simulink model "SSSC_PODcontrol"  (R2018a)
settings: Solver=ode23tb  StartTime=0  StopTime=5  MaxStep=1/60  RelTol=1e-4  AbsTol=1e-3
PreLoadFcn:
  | global Kp
  | global Tw
  | global T1
  | global T2
  | global T3
  | global T4
  | %--------------------------------------
  | global Kp1
  | global Tw1
  | global T11
  | global T21
  | global T31
  | global T41
  | %-------------------------------------
  | global Kp2
  | global Tw2
  | global T12
  | global T22
  | global T32
  | global T42
  | %-------------------------------------
InitFcn:
  | global Kp
  | global Tw
  | global T1
  | global T2
  | global T3
  | global T4
  | %--------------------------------------
  | global Kp1
  | global Tw1
  | global T11
  | global T21
  | global T31
  | global T41
  | %-------------------------------------
  | global Kp2
  | global Tw2
  | global T12
  | global T22
  | global T32
  | global T42
  | %-------------------------------------
values from neighbouring files (symbols this model uses):
  Kp = (x(1))    [fitnessfunc.m]
  Kp1 = (x(7))    [fitnessfunc.m]
  Kp2 = (x(13))    [fitnessfunc.m]
  T1 = best_Value(3)    [ACOMain.m]    (also in FPGA_POD_coefficients.mat = 0.46; Main.m; fitnessfunc.m = (x(3)); optimized_POD_parameters.mat = 0.46)
  T11 = (x(9))    [fitnessfunc.m]
  T12 = (x(15))    [fitnessfunc.m]
  T2 = best_Value(4)    [ACOMain.m]    (also in FPGA_POD_coefficients.mat = 0.49; Main.m; fitnessfunc.m = (x(4)); optimized_POD_parameters.mat = 0.49)
  T21 = (x(10))    [fitnessfunc.m]
  T22 = (x(16))    [fitnessfunc.m]
  T3 = best_Value(5)    [ACOMain.m]    (also in FPGA_POD_coefficients.mat = 0.32; Main.m; fitnessfunc.m = (x(5)); optimized_POD_parameters.mat = 0.32)
  T31 = (x(11))    [fitnessfunc.m]
  T32 = (x(17))    [fitnessfunc.m]
  T4 = best_Value(6)    [ACOMain.m]    (also in FPGA_POD_coefficients.mat = 0.1564; Main.m; fitnessfunc.m = (x(6)); optimized_POD_parameters.mat = 0.1564)
  T41 = (x(12))    [fitnessfunc.m]
  T42 = (x(18))    [fitnessfunc.m]
  Tw = best_Value(2)    [ACOMain.m]    (also in FPGA_POD_coefficients.mat = 10.1; Main.m; fitnessfunc.m = (x(2)); optimized_POD_parameters.mat = 10.1)
undefined symbols (not defined in the file or in its folder): D1, Delta
libraries: powerlib x21, powerlib_meascontrol x9, sps_avr x2, factslib x1
Description:
  | Copyright 2008-2018 The MathWorks, Inc.
settings Model: ExtModeAutoUpdateStatusClock=off  Creator=MathWorks  LastModifiedBy=Mehdi
settings SolverCC: AutoScaleAbsTol=off
settings DataIOCC: SaveFinalState=on  SaveFormat=Array  SignalLoggingSaveFormat=ModelDataLogs  SaveOutput=off  SaveTime=off  SignalLoggingName=sigsOut
settings OptimizationCC: BooleanDataType=off  ExpressionDepthLimit=2147483647  InitFltsAndDblsToZero=on  LifeSpan=inf
settings DebuggingCC: UnderspecifiedInitializationDetection=Classic  MergeDetectMultiDrivingBlocksExec=none  CheckExecutionContextPreStartOutputMsg=on  CheckExecutionContextRuntimeOutputMsg=on  SignalResolutionControl=TryResolveAllWithWarning  MultiTaskDSMMsg=warning  MultiTaskCondExecSysMsg=none  SigSpecEnsureSampleTimeMsg=none  FcnCallInpInsideContextMsg=warning  UnconnectedLineMsg=none  StateNameClashWarn=warning  SFUnexpectedBacktrackingDiag=warning  SFNoUnconditionalDefaultTransitionDiag=warning  SFExecutionAtInitializationDiag=none
settings HardwareCC: ProdBitPerPointer=32  ProdBitPerSizeT=32  ProdBitPerPtrDiffT=32  ProdLargestAtomicFloat=None  ProdIntDivRoundTo=Undefined  ProdEndianess=Unspecified  ProdWordSize=32  ProdHWDeviceType=32-bit Generic  TargetUnknown=on
settings ModelReferenceCC: PropagateSignalLabelsOutOfModel=off
settings CodeAppCC: StateflowObjectComments=on
settings GRTTargetCC: TargetLangStandard=C89/C90 (ANSI)  GeneratePreprocessorConditionals=Disable all  CombineOutputUpdateFcns=off  GRTInterface=on
settings ConfigComp: CovMetricSettings=dw  CovHtmlReporting=on  CovSaveCumulativeToWorkspaceVar=on  CovSaveSingleToWorkspaceVar=on  CovExternalEMLEnable=off  CovSFcnEnable=off
settings SimscapeCC: SimscapeNormalizeSystem=off

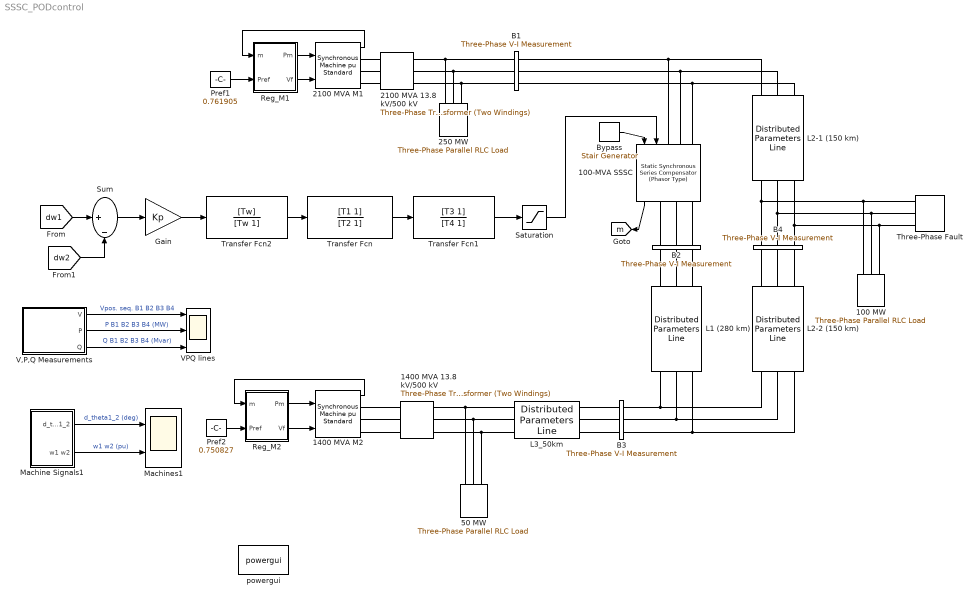
== system SSSC_PODcontrol ==
  100 MW : powerlib/Elements/Three-Phase Parallel RLC Load  LConnTagsString=A|B|C  Configuration=Y (grounded)  NominalVoltage=500e3  Vabc=[1e3 1e3 1e3]  Vabcp=[1e3 1e3 1e3]  NominalFrequency=60  UnbalancedPower=off  ActivePower=100e6  InductivePower=0  CapacitivePower=0  Pabc=[10e3 9e3 11e3]  QLabc=[100 90 110]  QCabc=[100 90 110]  Pabcp=[10e3 9e3 11e3]  QLabcp=[100 90 110]  QCabcp=[100 90 110]  Measurements=None  LoadType=constant Z
  100-MVA SSSC : factslib/Power-Electronics Based FACTS/Static Synchronous Series Compensator (Phasor Type)  SystemNominal=[ 500e3, 60 ]  SeriesNominal=[ 100e6, 0.1]  RL=[ 0.16/30, 0.16 ]  Iinit=[ 0 0]  VnomDC=40000  C_DC=375e-6  ExternalByPass=External control  Vqref=0.05  ExternalVqref=on  MaxRateVqRef=3  Par_VacReg=[0.03 1.5]/8  Par_VdcReg=[0.1e-3 20e-3]
      settings: SourceProductName=Simscape Power Systems  SourceProductBaseCode=PS
  1400 MVA M2 : powerlib/Machines/Synchronous Machine pu Standard  PresetModel=No  MechanicalLoad=Mechanical power Pm  ShowDetailedParameters=on  RotorType=Salient-pole  Units=per unit standard parameters  MeasurementBus=off  NominalParameters="[1400E6  13800   60 ]"  Reactances1=[ 31 32 33 34 35 36 37 ]  Reactances2=[ 1.305, 0.296, 0.252, 0.474, 0.243, 0.18 ]  dAxisTimeConstants=Short-circuit  qAxisTimeConstants=Open-circuit  TimeConstants1=[]  TimeConstants2=[]  TimeConstants3=[]  TimeConstants4=[]  TimeConstants5=[ 1.01, 0.053, 0.1 ]  TimeConstants6=[]  TimeConstants7=[]  TimeConstants8=[]  StatorResistance=2.8544e-3  Mechanical="[ 3.7 0  32]"  PolePairs=32  InitialConditions=[0 -71.2244 0.745111 0.745111 0.745111 -3.89206 -123.892 116.108 1.33295]  SetSaturation=off  Saturation=[0.6404,0.7127,0.8441,0.9214,0.9956,1.082,1.19,1.316,1.457;0.7,0.7698,0.8872,0.9466,0.9969,1.046,1.1,1.151,1.201]  LoadFlowParameters=[2 1000000000 13938 0 0]  TsPowergui=0  TsBlock=-1  IterativeModel=Forward Euler  IterativeDiscreteModel=Trapezoidal non iterative  BusType=PV  Pref=0  Qref=0  Qmin=-inf  Qmax=inf  PLF=0  QLF=0
      settings: AttributesFormatString=\n\n  SourceProductName=Simscape Power Systems
  1400 MVA 13.8 kV/500 kV : powerlib/Elements/Three-Phase Transformer (Two Windings)  Winding1Connection=Delta (D1)  Winding2Connection=Yg  CoreType=Three single-phase transformers  SetSaturation=off  Hysteresis=off  DataFile='basic_model'  SetInitialFlux=off  Measurements=None  UNITS=pu  NominalPower=[ 1400e6 60 ]  Winding1="[ 13.8e3 0.002  0.0]"  Winding2=[ 500e3 0.002 0.12]  Rm=500  Lm=500  L0=0.5  Saturation="[ 0,0  ;  0.005,1.2  ;  1.0,1.4 ]"  InitialFluxes=[ 0.8 , -0.8 , 0.7 ]  MoreParameters=off  BreakLoop=off  DataType=off  TransfoNumber=0
  2100 MVA M1 : powerlib/Machines/Synchronous Machine pu Standard  PresetModel=No  MechanicalLoad=Mechanical power Pm  ShowDetailedParameters=on  RotorType=Salient-pole  Units=per unit standard parameters  MeasurementBus=off  NominalParameters="[2100E6  13800   60 ]"  Reactances1=[ 31 32 33 34 35 36 37 ]  Reactances2=[ 1.305, 0.296, 0.252, 0.474, 0.243, 0.18 ]  dAxisTimeConstants=Short-circuit  qAxisTimeConstants=Open-circuit  TimeConstants1=[]  TimeConstants2=[]  TimeConstants3=[]  TimeConstants4=[]  TimeConstants5=[ 1.01, 0.053, 0.1 ]  TimeConstants6=[]  TimeConstants7=[]  TimeConstants8=[]  StatorResistance=2.8544e-3  Mechanical="[ 3.7 0  32]"  PolePairs=32  InitialConditions=[0 -58.9841 0.763417 0.763417 0.763417 14.3746 -105.625 134.375 1.2256]  SetSaturation=off  Saturation=[0.6404,0.7127,0.8441,0.9214,0.9956,1.082,1.19,1.316,1.457;0.7,0.7698,0.8872,0.9466,0.9969,1.046,1.1,1.151,1.201]  LoadFlowParameters=[1 1600000000 0 0 0]  TsPowergui=0  TsBlock=-1  IterativeModel=Forward Euler  IterativeDiscreteModel=Trapezoidal non iterative  BusType=PV  Pref=0  Qref=0  Qmin=-inf  Qmax=inf  PLF=0  QLF=0
      settings: AttributesFormatString=\n\n  SourceProductName=Simscape Power Systems
  2100 MVA 13.8 kV/500 kV : powerlib/Elements/Three-Phase Transformer (Two Windings)  Winding1Connection=Delta (D1)  Winding2Connection=Yg  CoreType=Three single-phase transformers  SetSaturation=off  Hysteresis=off  DataFile='basic_model'  SetInitialFlux=off  Measurements=None  UNITS=pu  NominalPower=[ 2100e6 60 ]  Winding1="[ 13.8e3 0.002  0.0]"  Winding2=[ 500e3 0.002 0.12]  Rm=500  Lm=500  L0=0.5  Saturation="[ 0,0  ;  0.005,1.2  ;  1.0,1.4 ]"  InitialFluxes=[ 0.8 , -0.8 , 0.7 ]  MoreParameters=off  BreakLoop=off  DataType=off  TransfoNumber=0
  250 MW : powerlib/Elements/Three-Phase Parallel RLC Load  LConnTagsString=A|B|C  Configuration=Y (grounded)  NominalVoltage=500e3  Vabc=[1e3 1e3 1e3]  Vabcp=[1e3 1e3 1e3]  NominalFrequency=60  UnbalancedPower=off  ActivePower=250e6  InductivePower=0  CapacitivePower=0  Pabc=[10e3 9e3 11e3]  QLabc=[100 90 110]  QCabc=[100 90 110]  Pabcp=[10e3 9e3 11e3]  QLabcp=[100 90 110]  QCabcp=[100 90 110]  Measurements=None  LoadType=constant Z
  50 MW : powerlib/Elements/Three-Phase Parallel RLC Load  LConnTagsString=A|B|C  Configuration=Y (grounded)  NominalVoltage=500e3  Vabc=[1e3 1e3 1e3]  Vabcp=[1e3 1e3 1e3]  NominalFrequency=60  UnbalancedPower=off  ActivePower=50e6  InductivePower=0  CapacitivePower=0  Pabc=[10e3 9e3 11e3]  QLabc=[100 90 110]  QCabc=[100 90 110]  Pabcp=[10e3 9e3 11e3]  QLabcp=[100 90 110]  QCabcp=[100 90 110]  Measurements=None  LoadType=constant Z
  B1 : powerlib/Measurements/Three-Phase V-I Measurement  VoltageMeasurement=phase-to-ground  SetLabelV=on  LabelV=Vabc_B1  Vpu=on  VpuLL=off  CurrentMeasurement=yes  SetLabelI=on  LabelI=Iabc_B1  Ipu=on  Pbase=100e6  Vbase=500e3  OutputType=Complex  PhasorSimulation=on  PSBequivalent=0
  B2 : powerlib/Measurements/Three-Phase V-I Measurement  VoltageMeasurement=phase-to-ground  SetLabelV=on  LabelV=Vabc_B2  Vpu=on  VpuLL=off  CurrentMeasurement=yes  SetLabelI=on  LabelI=Iabc_B2  Ipu=on  Pbase=100e6  Vbase=500e3  OutputType=Complex  PhasorSimulation=on  PSBequivalent=0
  B3 : powerlib/Measurements/Three-Phase V-I Measurement  VoltageMeasurement=phase-to-ground  SetLabelV=on  LabelV=Vabc_B3  Vpu=on  VpuLL=off  CurrentMeasurement=yes  SetLabelI=on  LabelI=Iabc_B3  Ipu=on  Pbase=100e6  Vbase=500e3  OutputType=Complex  PhasorSimulation=on  PSBequivalent=0
  B4 : powerlib/Measurements/Three-Phase V-I Measurement  VoltageMeasurement=phase-to-ground  SetLabelV=on  LabelV=Vabc_B4  Vpu=on  VpuLL=off  CurrentMeasurement=yes  SetLabelI=on  LabelI=Iabc_B4  Ipu=on  Pbase=100e6  Vbase=500e3  OutputType=Complex  PhasorSimulation=on  PSBequivalent=0
  Bypass : powerlib_meascontrol/Pulse & Signal Generators/Stair Generator  t=[0, 0.1]  e=[1, 0 ]  Ts=0
      settings: SourceProductName=Simscape Power Systems
  Gain : Gain  Gain=Kp
  L1 (280 km) : powerlib/Elements/Distributed Parameters Line  Phases=3  Frequency=60  Resistance=[0.01273*2 0.3864]  Inductance="[0.9337e-3  4.1264e-3]"  Capacitance=[12.74e-9 7.751e-9]  Length=280  x1=[8.57453623118534e-09 1498726.92101237 1498731.61187745;376.991118430775 376.991118430775 376.991118430775;-0.207010743951092 -0.27921503857041 -1.85001560704433]  x2=[3.70968821408053e-08 1547199.03240546 1547203.81684282;376.991118430775 376.991118430775 376.991118430775;-1.73289441680718 -0.258096765893564 -1.8288976303327]  x3=[7.34085838580846e-11 5978.20234022193 5978.21644518815;376.991118430775 376.991118430775 376.991118430775;3.00344553485436 -0.528094897252935 -2.09889563309672]  x4=[8.19150865277484e-11 5275.11122531886 5275.13210158224;376.991118430775 376.991118430775 376.991118430775;-0.77313679488924 -0.365166148081062 -1.93596698668438]  x5=0.00158351638758808  V1=ones(3,3)  V2=ones(3,3)  I1=ones(3,3)  I2=ones(3,3)  nHarmo=1  Measurements=None
      settings: AttributesFormatString=\n  SourceProductName=Simscape Power Systems
  L2-1 (150 km) : powerlib/Elements/Distributed Parameters Line  Phases=3  Frequency=60  Resistance=[0.01273*2 0.3864]  Inductance="[0.9337e-3  4.1264e-3]"  Capacitance=[12.74e-9 7.751e-9]  Length=150  x1=[8.14603489907096e-09 1498726.88392124 1498731.57478671;376.991118430775 376.991118430775 376.991118430775;-1.17916675081451 -0.110185299814799 -1.68098586828873]  x2=[1.43076082998811e-07 1551001.48715857 1551006.3144557;376.991118430775 376.991118430775 376.991118430775;-1.56135800434571 -0.111564642343529 -1.68236536135358]  x3=[5.49715704458232e-10 5715.20612101038 5715.21968310763;376.991118430775 376.991118430775 376.991118430775;-2.89588916944808 -0.380270362847911 -1.95107110411091]  x4=[5.12825351090249e-10 5653.45328530216 5653.47513824224;376.991118430775 376.991118430775 376.991118430775;-0.12404020965703 -0.0353350035895054 -1.60613581272854]  x5=0.000848312350493614  V1=ones(3,3)  V2=ones(3,3)  I1=ones(3,3)  I2=ones(3,3)  nHarmo=1  Measurements=None
      settings: AttributesFormatString=\n  SourceProductName=Simscape Power Systems
  L2-2 (150 km) : powerlib/Elements/Distributed Parameters Line  Phases=3  Frequency=60  Resistance=[0.01273*2 0.3864]  Inductance="[0.9337e-3  4.1264e-3]"  Capacitance=[12.74e-9 7.751e-9]  Length=150  x1=[1.43076082998811e-07 1551001.48715857 1551006.3144557;376.991118430775 376.991118430775 376.991118430775;-1.56135800434571 -0.111564642343529 -1.68236536135358]  x2=[3.70968821408053e-08 1547199.03240546 1547203.81684282;376.991118430775 376.991118430775 376.991118430775;-1.45572902458812 -0.0890671266930067 -1.65986799113215]  x3=[4.05230677949172e-10 6333.0550295995 6333.07045412649;376.991118430775 376.991118430775 376.991118430775;-0.243158405131011 -0.179600649437888 -1.75040138546907]  x4=[4.4859545811629e-10 5046.70981789123 5046.72971787752;376.991118430775 376.991118430775 376.991118430775;-2.82744541099243 -0.221522382170995 -1.79232320866502]  x5=0.000848312350493614  V1=ones(3,3)  V2=ones(3,3)  I1=ones(3,3)  I2=ones(3,3)  nHarmo=1  Measurements=None
      settings: AttributesFormatString=\n  SourceProductName=Simscape Power Systems
  L3_50km : powerlib/Elements/Distributed Parameters Line  Phases=3  Frequency=60  Resistance=[0.01273*2 0.3864]  Inductance="[0.9337e-3  4.1264e-3]"  Capacitance=[12.74e-9 7.751e-9]  Length=50  x1=[3.70968821408053e-08 1547199.03240546 1547203.81684282;376.991118430775 376.991118430775 376.991118430775;-1.2425248767273 0.0409556726920371 -1.5298451917471]  x2=[1.70902936205603e-09 1523504.65927186 1523509.34411468;376.991118430775 376.991118430775 376.991118430775;-0.382562555915443 0.0539283570396382 -1.51687260959561]  x3=[4.3479436689631e-10 6826.59857622228 6826.61106408169;376.991118430775 376.991118430775 376.991118430775;0.404606683004551 0.223538538849403 -1.34726198288477]  x4=[4.43312318202334e-10 4841.29117916682 4841.31490602355;376.991118430775 376.991118430775 376.991118430775;-2.61441187928109 -0.281614140729434 -1.85241468519146]  x5=0.000282770783497871  V1=ones(3,3)  V2=ones(3,3)  I1=ones(3,3)  I2=ones(3,3)  nHarmo=1  Measurements=None
      settings: AttributesFormatString=\n  SourceProductName=Simscape Power Systems
  Machine Signals1 : Subsystem
  Machines1 : Scope  NumInputPorts=2
  Pref1 : Constant  Value=0.761905
  Pref2 : Constant  Value=0.750827
  Reg_M1 : Subsystem
  Reg_M2 : Subsystem
  Saturation : Saturate  UpperLimit=0.15  LowerLimit=-0.15
  Sum : Sum  Inputs=|+-
  Three-Phase Fault : powerlib/Elements/Three-Phase Fault  InitialStates=0  FaultA=off  FaultB=off  FaultC=off  GroundFault=on  SwitchTimes=[ 20/60 30/60]+1  External=off  SwitchStatus=NaN  FaultResistance=0.001  GroundResistance=0.001  SnubberResistance=1e6  SnubberCapacitance=inf  Measurements=None
  Transfer Fcn : TransferFcn  Numerator=[T1 1]  Denominator=[T2 1]
  Transfer Fcn1 : TransferFcn  Numerator=[T3 1]  Denominator=[T4 1]
  Transfer Fcn2 : TransferFcn  Numerator=[Tw]  Denominator=[Tw 1]
  V,P,Q Measurements : Subsystem
      mask Display: disp('V P Q\nMeasurements')
  VPQ lines : Scope  NumInputPorts=3
  powergui : powerlib/powergui  Priority=2  SimulationMode=Phasor  SampleTime=0  frequency=60  Iterations=50  frequencyindice=60  Pbase=100e6  ErrMax=1e-4  UnitsV=kV  UnitsW=MW  buscounter=0  FunctionMessages=off  echomessages=off  EnableUseOfTLC=off  CurrentSourceSwitches=off  DisableSnubberDevices=off  DisableRonSwitches=off  DisableVfSwitches=off  DisplayEquations=off  SolverType=Tustin  Interpol=off  ExternalGateDelay=off  methode=off  Ts=0  x0status=blocks  SPID=off  SwTol=0  HookPort=off  RestoreLinks=warning  ResistiveCurrentMeasurement=off  Frange=[0:2:500]  Ylog=off  Xlog=on  ShowGrid=off  save=off  variable=ZData  structure=0  ZoomFFT=on  StartTime=0.0  cycles=1  DisplayStyle=1  fundamental=60  FreqAxis=off  MaxFrequency=1000  frequencyindicesteady=1  RmsSteady=1  display=off
  tag scope: m=global
  wires:
  Reg_M1/1(Pm) -> 2100 MVA M1/1
  Reg_M1/2(Vf) -> 2100 MVA M1/2
  Pref1/1 -> Reg_M1/2(Pref)
  2100 MVA M1/1 -> Reg_M1/1(m)
  Reg_M2/1(Pm) -> 1400 MVA M2/1
  Reg_M2/2(Vf) -> 1400 MVA M2/2
  Pref2/1 -> Reg_M2/2(Pref)
  1400 MVA M2/1 -> Reg_M2/1(m)
  100-MVA SSSC/1 -> [m]
  Bypass/1 -> 100-MVA SSSC/1
  Transfer Fcn/1 -> Transfer Fcn1/1
  Gain/1 -> Transfer Fcn2/1
  Transfer Fcn2/1 -> Transfer Fcn/1
  Sum/1 -> Gain/1
  [dw2] -> Sum/2
  [dw1] -> Sum/1
  Transfer Fcn1/1 -> Saturation/1
  Saturation/1 -> 100-MVA SSSC/2
  V,P,Q Measurements/3(Q) -> VPQ lines/3  "Q B1 B2 B3 B4 (Mvar)"
  V,P,Q Measurements/2(P) -> VPQ lines/2  "P B1 B2 B3 B4 (MW)"
  Machine Signals1/2(w1 w2) -> Machines1/2  "w1 w2 (pu)"
  V,P,Q Measurements/1(V) -> VPQ lines/1  "Vpos. seq. B1 B2 B3 B4"
  Machine Signals1/1(d_theta1_2) -> Machines1/1  "d_theta1_2 (deg)"
  connections:
  2100 MVA M1/RConn1 -- 2100 MVA 13.8 kV/500 kV/LConn1
  2100 MVA M1/RConn2 -- 2100 MVA 13.8 kV/500 kV/LConn2
  2100 MVA M1/RConn3 -- 2100 MVA 13.8 kV/500 kV/LConn3
  250 MW/LConn1 -- 2100 MVA 13.8 kV/500 kV/RConn1 -- B1/LConn1
  250 MW/LConn2 -- 2100 MVA 13.8 kV/500 kV/RConn2 -- B1/LConn2
  250 MW/LConn3 -- 2100 MVA 13.8 kV/500 kV/RConn3 -- B1/LConn3
  100-MVA SSSC/LConn1 -- B1/RConn1 -- L2-1 (150 km)/LConn1
  100-MVA SSSC/LConn2 -- B1/RConn2 -- L2-1 (150 km)/LConn2
  100-MVA SSSC/LConn3 -- B1/RConn3 -- L2-1 (150 km)/LConn3
  1400 MVA M2/RConn1 -- 1400 MVA 13.8 kV/500 kV/LConn1
  1400 MVA M2/RConn2 -- 1400 MVA 13.8 kV/500 kV/LConn2
  1400 MVA M2/RConn3 -- 1400 MVA 13.8 kV/500 kV/LConn3
  B3/RConn1 -- L2-2 (150 km)/RConn1 -- L1 (280 km)/RConn1
  B3/RConn2 -- L2-2 (150 km)/RConn2 -- L1 (280 km)/RConn2
  B3/RConn3 -- L1 (280 km)/RConn3 -- L2-2 (150 km)/RConn3
  B4/RConn1 -- L2-2 (150 km)/LConn1
  B4/RConn2 -- L2-2 (150 km)/LConn2
  B4/RConn3 -- L2-2 (150 km)/LConn3
  Three-Phase Fault/LConn1 -- B4/LConn1 -- L2-1 (150 km)/RConn1 -- 100 MW/LConn1
  Three-Phase Fault/LConn2 -- B4/LConn2 -- L2-1 (150 km)/RConn2 -- 100 MW/LConn2
  Three-Phase Fault/LConn3 -- B4/LConn3 -- L2-1 (150 km)/RConn3 -- 100 MW/LConn3
  1400 MVA 13.8 kV/500 kV/RConn1 -- L3_50km/RConn1 -- 50 MW/LConn1
  1400 MVA 13.8 kV/500 kV/RConn2 -- L3_50km/RConn2 -- 50 MW/LConn2
  1400 MVA 13.8 kV/500 kV/RConn3 -- L3_50km/RConn3 -- 50 MW/LConn3
  100-MVA SSSC/RConn1 -- B2/LConn1
  100-MVA SSSC/RConn2 -- B2/LConn2
  100-MVA SSSC/RConn3 -- B2/LConn3
  B2/RConn1 -- L1 (280 km)/LConn1
  B2/RConn2 -- L1 (280 km)/LConn2
  B2/RConn3 -- L1 (280 km)/LConn3
  L3_50km/LConn1 -- B3/LConn1
  L3_50km/LConn2 -- B3/LConn2
  L3_50km/LConn3 -- B3/LConn3

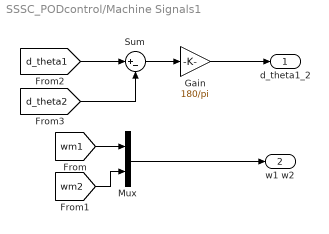
== system SSSC_PODcontrol/Machine Signals1 ==
  Gain : Gain  Gain=180/pi  SaturateOnIntegerOverflow=on  OutDataTypeStr=Inherit: Same as input  ParamDataTypeStr=Inherit: Same as input
  Mux : Mux  Inputs=2
  Sum : Sum  Inputs=|+-  SaturateOnIntegerOverflow=on  InputSameDT=on  OutDataTypeStr=Inherit: Same as first input
  d_theta1_2 : Outport
  w1 w2 : Outport  Port=2
  wires:
  Sum/1 -> Gain/1
  [d_theta1] -> Sum/1
  [wm1] -> Mux/1
  Mux/1 -> w1 w2/1
  Gain/1 -> d_theta1_2/1
  [wm2] -> Mux/2
  [d_theta2] -> Sum/2

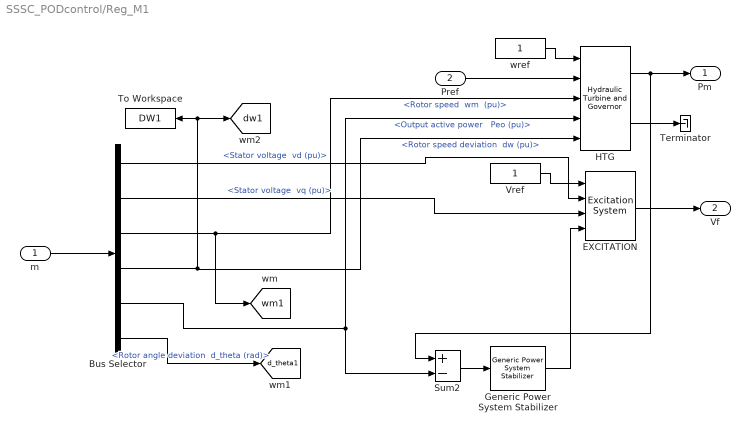
== system SSSC_PODcontrol/Reg_M1 ==
  m : Inport
  Pref : Inport  Port=2
  Bus Selector : BusSelector  OutputSignals="dq0 components.Stator voltage  vd (pu),dq0 components.Stator voltage  vq (pu),Mechanical.Rotor speed  wm  (pu),Mechanical.Rotor speed deviation  dw (pu),Output active power   Peo (pu),Mechanical.Rotor angle deviation  d_theta (rad)"
  EXCITATION : sps_avr/Excitation System  tr=20e-3  reg=[ 200, 0.001 ]  exc=[ 1, 0 ]  tgr=[ 0, 0 ]  damp=[ 0.001, 0.1 ]  sat=[ 0, 0 ]  lim="[ 0,  7, 0 ]"  v0=[1,1.2256]
      settings: SourceProductName=Simscape Power Systems  SourceProductBaseCode=PS
  Generic Power System Stabilizer : powerlib/Machines/Generic Power System Stabilizer  Tsensor=15e-3  K=Kp1  Twashout=Tw1  Tleadlag1=[T11 T21]  Tleadlag2="[T31  T41]"  VSlimits=[-0.15 0.15]  Vinit=0  Plot_On=off  MagdB_On=on  FreqRange=logspace(-2,2,500)
      settings: SourceProductName=Simscape Power Systems  SourceProductBaseCode=PS
  HTG : powerlib/Machines/Hydraulic Turbine and Governor  sm="[ 10/3  0.07 ]"  gate="[  0.01  0.97518  -0.1  0.1 ]"  reg="[  0.05  1.163  0.105  0  0.01  ]"  hyd="[  0  2.67  ]"  dref=0  po=0.763568
      settings: SourceProductName=Simscape Power Systems  SourceProductBaseCode=PS
  Sum2 : Sum  Inputs=+-  SaturateOnIntegerOverflow=on  InputSameDT=on  OutDataTypeStr=Inherit: Same as first input
  Terminator : Terminator
  To Workspace : ToWorkspace  VariableName=DW1  SampleTime=-1
  Vref : Constant
  wref : Constant
  Pm : Outport  InitialOutput=0
  Vf : Outport  Port=2  InitialOutput=0
  tag scope: d_theta1=global, dw1=global, wm1=global
  wires:
  Sum2/1 -> Generic Power System Stabilizer/1
  Bus Selector/1 -> EXCITATION/2  "<Stator voltage  vd (pu)>"
  EXCITATION/1 -> Vf/1
  Bus Selector/2 -> EXCITATION/3  "<Stator voltage  vq (pu)>"
  HTG/1 -> Sum2/1, Pm/1
  wref/1 -> HTG/1
  Pref/1 -> HTG/2
  Bus Selector/3 -> [wm1], HTG/3  "<Rotor speed  wm  (pu)>"
  Bus Selector/5 -> HTG/4, Sum2/2  "<Output active power   Peo (pu)>"
  Bus Selector/4 -> HTG/5, To Workspace/1, [dw1]  "<Rotor speed deviation  dw (pu)>"
  m/1 -> Bus Selector/1
  Vref/1 -> EXCITATION/1
  HTG/2 -> Terminator/1
  Generic Power System Stabilizer/1 -> EXCITATION/4
  Bus Selector/6 -> [d_theta1]  "<Rotor angle deviation  d_theta (rad)>"

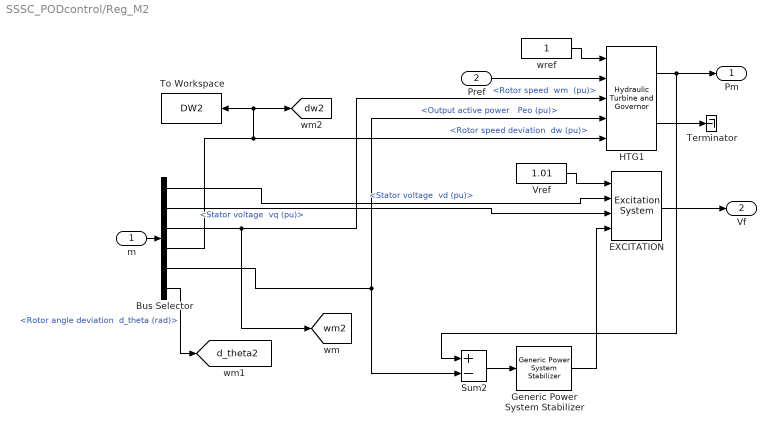
== system SSSC_PODcontrol/Reg_M2 ==
  m : Inport
  Pref : Inport  Port=2
  Bus Selector : BusSelector  OutputSignals="dq0 components.Stator voltage  vd (pu),dq0 components.Stator voltage  vq (pu),Mechanical.Rotor speed  wm  (pu),Mechanical.Rotor speed deviation  dw (pu),Output active power   Peo (pu),Mechanical.Rotor angle deviation  d_theta (rad)"
  EXCITATION : sps_avr/Excitation System  tr=20e-3  reg=[ 200, 0.001 ]  exc=[ 1, 0 ]  tgr=[ 0, 0 ]  damp=[ 0.001, 0.1 ]  sat=[ 0, 0 ]  lim="[ 0,  7, 0 ]"  v0=[1.01,1.33295]
      settings: SourceProductName=Simscape Power Systems  SourceProductBaseCode=PS
  Generic Power System Stabilizer : powerlib/Machines/Generic Power System Stabilizer  Tsensor=15e-3  K=Kp2  Twashout=Tw2  Tleadlag1="[T12  T22]"  Tleadlag2="[T32  T42]"  VSlimits=[-0.15 0.15]  Vinit=0  Plot_On=off  MagdB_On=on  FreqRange=logspace(-2,2,500)
      settings: SourceProductName=Simscape Power Systems  SourceProductBaseCode=PS
  HTG1 : powerlib/Machines/Hydraulic Turbine and Governor  sm="[ 10/3  0.07 ]"  gate="[  0.01  0.97518  -0.1  0.1 ]"  reg="[  0.05  1.163  0.105  0  0.01  ]"  hyd="[  0  2.67  ]"  dref=0  po=0.752412
      settings: SourceProductName=Simscape Power Systems  SourceProductBaseCode=PS
  Sum2 : Sum  Inputs=+-  SaturateOnIntegerOverflow=on  InputSameDT=on  OutDataTypeStr=Inherit: Same as first input
  Terminator : Terminator
  To Workspace : ToWorkspace  VariableName=DW2  SampleTime=-1
  Vref : Constant  Value=1.01
  wref : Constant
  Pm : Outport  InitialOutput=0
  Vf : Outport  Port=2  InitialOutput=0
  tag scope: d_theta2=global, dw2=global, wm2=global
  wires:
  HTG1/2 -> Terminator/1
  Vref/1 -> EXCITATION/1
  m/1 -> Bus Selector/1
  Bus Selector/4 -> HTG1/5, [dw2], To Workspace/1  "<Rotor speed deviation  dw (pu)>"
  Bus Selector/5 -> Sum2/2, HTG1/4  "<Output active power   Peo (pu)>"
  Bus Selector/3 -> [wm2], HTG1/3  "<Rotor speed  wm  (pu)>"
  Pref/1 -> HTG1/2
  wref/1 -> HTG1/1
  HTG1/1 -> Pm/1, Sum2/1
  Bus Selector/2 -> EXCITATION/3  "<Stator voltage  vq (pu)>"
  EXCITATION/1 -> Vf/1
  Bus Selector/1 -> EXCITATION/2  "<Stator voltage  vd (pu)>"
  Sum2/1 -> Generic Power System Stabilizer/1
  Generic Power System Stabilizer/1 -> EXCITATION/4
  Bus Selector/6 -> [d_theta2]  "<Rotor angle deviation  d_theta (rad)>"

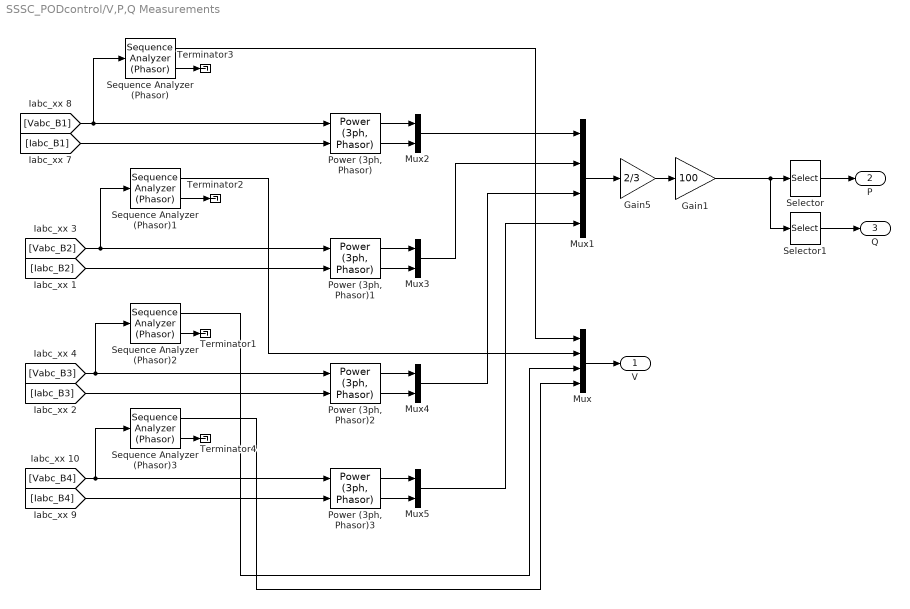
== system SSSC_PODcontrol/V,P,Q Measurements ==
  Gain1 : Gain  Gain=100  SaturateOnIntegerOverflow=on  OutDataTypeStr=Inherit: Same as input  ParamDataTypeStr=Inherit: Same as input
  Gain5 : Gain  Gain=2/3  SaturateOnIntegerOverflow=on  OutDataTypeStr=Inherit: Same as input  ParamDataTypeStr=Inherit: Same as input
  Mux : Mux
  Mux1 : Mux
  Mux{2..5} (4 alike) : Mux  Inputs=2
  Power (3ph, Phasor){,1..3} (4 alike) : powerlib_meascontrol/Measurements/Power (3ph, Phasor)
      settings: SourceProductName=Simscape Power Systems  SourceProductBaseCode=PS
  Selector : Selector  InputPortWidth=8  IndexOptions=Index vector (dialog)  Indices=[1 3 5 7 ]  OutputSizes=1
  Selector1 : Selector  InputPortWidth=8  IndexOptions=Index vector (dialog)  Indices=[1 3 5 7 ]+1  OutputSizes=1
  Sequence Analyzer (Phasor){,1..3} (4 alike) : powerlib_meascontrol/Measurements/Sequence Analyzer (Phasor)  seq=Positive
      settings: SourceProductName=Simscape Power Systems  SourceProductBaseCode=PS
  Terminator{1..4} (4 alike) : Terminator
  V : Outport
  P : Outport  Port=2
  Q : Outport  Port=3
  wires:
  Gain1/1 -> Selector/1, Selector1/1
  Gain5/1 -> Gain1/1
  Sequence Analyzer (Phasor)1/2 -> Terminator2/1
  [Vabc_B2] -> "Power (3ph, Phasor)1"/1, Sequence Analyzer (Phasor)1/1
  [Iabc_B2] -> "Power (3ph, Phasor)1"/2
  [Vabc_B3] -> "Power (3ph, Phasor)2"/1, Sequence Analyzer (Phasor)2/1
  [Iabc_B3] -> "Power (3ph, Phasor)2"/2
  Sequence Analyzer (Phasor)2/2 -> Terminator1/1
  Sequence Analyzer (Phasor)1/1 -> Mux/2
  Sequence Analyzer (Phasor)2/1 -> Mux/3
  Mux/1 -> V/1
  Mux1/1 -> Gain5/1
  Selector/1 -> P/1
  Selector1/1 -> Q/1
  Sequence Analyzer (Phasor)3/2 -> Terminator4/1
  Sequence Analyzer (Phasor)3/1 -> Mux/4
  Sequence Analyzer (Phasor)/1 -> Mux/1
  [Vabc_B1] -> "Power (3ph, Phasor)"/1, Sequence Analyzer (Phasor)/1
  [Iabc_B1] -> "Power (3ph, Phasor)"/2
  "Power (3ph, Phasor)"/2 -> Mux2/2
  "Power (3ph, Phasor)"/1 -> Mux2/1
  Mux2/1 -> Mux1/1
  Mux3/1 -> Mux1/2
  "Power (3ph, Phasor)1"/1 -> Mux3/1
  "Power (3ph, Phasor)1"/2 -> Mux3/2
  "Power (3ph, Phasor)2"/1 -> Mux4/1
  "Power (3ph, Phasor)2"/2 -> Mux4/2
  Mux4/1 -> Mux1/3
  [Vabc_B4] -> "Power (3ph, Phasor)3"/1, Sequence Analyzer (Phasor)3/1
  [Iabc_B4] -> "Power (3ph, Phasor)3"/2
  "Power (3ph, Phasor)3"/1 -> Mux5/1
  "Power (3ph, Phasor)3"/2 -> Mux5/2
  Mux5/1 -> Mux1/4
  Sequence Analyzer (Phasor)/2 -> Terminator3/1
